simulink model "Pid_Basic"  (R2024b)
settings: Solver=VariableStepAuto  StartTime=0.0  StopTime=10.0  RelTol=1e-3
settings Model: Creator=vishwanth  LastModifiedBy=vishwanth

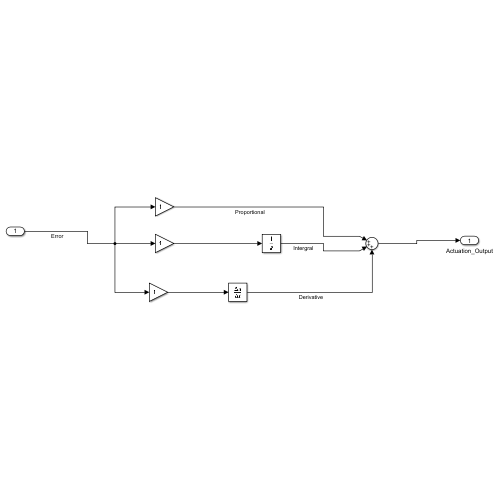
[thumbnail: Simulink's stored preview of the top-level diagram]
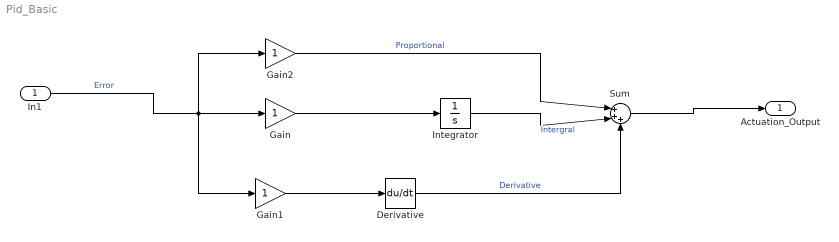
== system Pid_Basic ==
  In1 : Inport
  Derivative : Derivative
  Gain : Gain
  Gain1 : Gain
  Gain2 : Gain
  Integrator : Integrator
  Sum : Sum  Inputs=|+++
  Actuation_Output : Outport
  wires:
  Gain1/1 -> Derivative/1
  Gain/1 -> Integrator/1
  In1/1 -> Gain1/1, Gain2/1, Gain/1  "Error"
  Gain2/1 -> Sum/1  "Proportional"
  Integrator/1 -> Sum/2  "Intergral"
  Derivative/1 -> Sum/3  "Derivative"
  Sum/1 -> Actuation_Output/1
